simulink model "a2024_V2X_6V_Simulink_model"  (R2023b)
settings: Solver=VariableStepAuto  StartTime=0.0  StopTime=30  MaxStep=1e-2  RelTol=1e-3  AbsTol=1e-3
values from neighbouring files (symbols this model uses):
  b = 1.6    [a2024_v2x_matlab_6veh.m]
  mEgo = 1500    [a2024_v2x_matlab_6veh.m]
  Mode = 1    [a2024_v2x_matlab_6veh.m]    (also in v2x_matlab.m; v2x_matlabV2.m; v2x_matlab_6veh.m; v2x_matlab_R.m)
  pilot = (randi(s,[0 1],pilotsPerSym,1)-0.5)*2    [v2x_matlab.m]
  RxPowerV1 = zeros(sizeEgoWP+2, sizeV1WP+2)    [a2024_v2x_matlab_6veh.m]
  RxPowerV2 = zeros(sizeEgoWP+2, sizeV2WP+2)    [a2024_v2x_matlab_6veh.m]
  RxPowerV3 = zeros(sizeEgoWP+2, sizeV3WP+2)    [a2024_v2x_matlab_6veh.m]
  RxPowerV4 = zeros(sizeEgoWP+2, sizeV4WP+2)    [a2024_v2x_matlab_6veh.m]
  RxPowerV5 = zeros(sizeEgoWP+2, sizeV5WP+2)    [a2024_v2x_matlab_6veh.m]
  RxPowerV6 = zeros(sizeEgoWP+2, sizeV6WP+2)    [a2024_v2x_matlab_6veh.m]
  sampleTime = 0.1    [a2024_v2x_matlab_6veh.m]    (also in v2x_matlab.m; v2x_matlabV2.m; v2x_matlab_6veh.m; v2x_matlab_R.m)
  t_gap = 1.4    [a2024_v2x_matlab_6veh.m]
  waypoints = [egoWP(:,2) egoWP(:,1), zeroforwp]    [a2024_v2x_matlab_6veh.m]    (also in misc.m = data.data.ActorSpecifications(1,1).Waypoints(:,[1,2]); v2x_matlab.m = data.data.ActorSpecifications(1,1).Waypoints(:,[1,2]); v2x_matlabV2.m = [5 -1.6 0; v2x_matlab_R.m = [5 -1.6 0)
  ZeroActors = struct(     'ActorID',0,     'Position', [1000 1000 1000],      'Velocity', [0 0 0],      'Roll', 0,      'Pitch', 0,      'Yaw', 0,      'AngularVelocity', [0 0 0])    [v2x_matlabV2.m]    (also in v2x_matlab_R.m)
undefined symbols (not defined in the file or in its folder): driving, PredictionHorizon, Ts
libraries: commofdm x50, commcnvcod2 x39, simulink x34, commdigbbndam3 x31, commblkintrlv2 x26, commdigbbndpm3 x14, simulink_extras x12, drivingscenarioandsensors x3, mpcadaslib x2, commchan3 x1, vehdynlibdriver x1, commrandsrc3 x1
(part 1 of 6)
settings Model: DataDictionary=V2X.sldd  PacingRate=2  Creator=Fauszt Gábor  LastModifiedBy=Fauszt Gábor

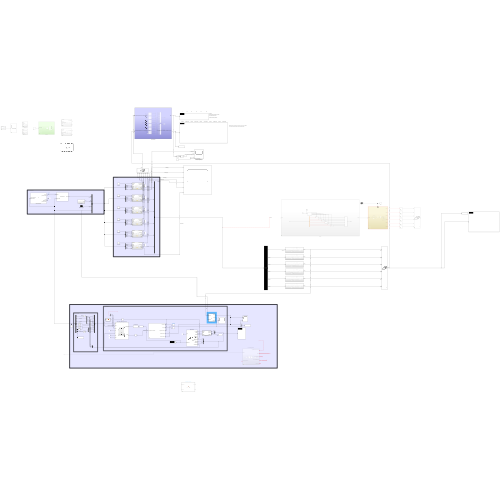
[thumbnail: Simulink's stored preview of the top-level diagram]
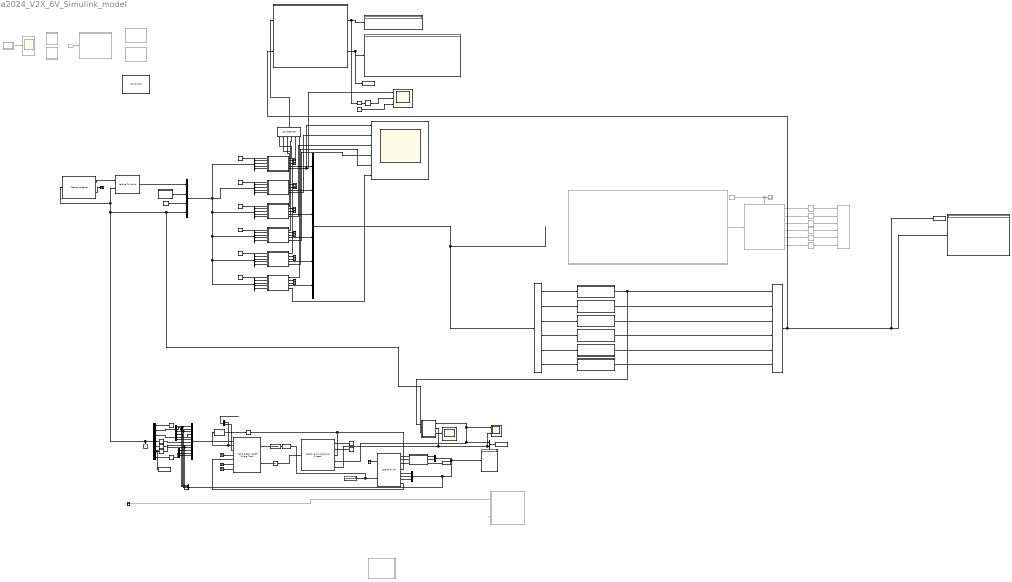
== system a2024_V2X_6V_Simulink_model ==
  note: ACC
  note: Display block can show only the first 10 columns of a matrix
      | thus, the columns of the 6th vehicle cannot be seen.
  note: V1 Received
  note: V1 Sent
  note: All packets sent' counter
  note: Received correct packets' counter
  note: PDR [%]
  note: V2
  note: V1
  note: Subsystem3
  note: Scenario Reader
  note: V3
  note: V4
  note: V5
  note: V6
  note: V2 Received
  note: V2 Sent
  note: V3 Received
  note: V3 Sent
  note: V4 Received
  note: V4 Sent
  note: V5 Received
  note: V5 Sent
  note: PDR of the last 20 packets
  note: Pack Ego Actor
  note: Ego Dynamics
  1/2 QPSK SNR és PDR a campus forgatókönyvre : Scope  NumInputPorts=3
  Adaptive Cruise Control System1 : mpcadaslib/Adaptive Cruise Control System  EgoModel=tf(1,[0.5,1,0])  InitialEgoVelocity=12  DefaultSpacing=0  MaxVelocity=20  MinAcceleration=-2  amin_ext=off  MaxAcceleration=4  amax_ext=off  Ts=0.01  PredictionHorizon=3  ControllerBehavior=0.950  suboptimal=off  maxiter=10  datatypeopt=double  optmode=off  trackmode=off
      settings: LibrarySourceBlock=mpclib/Automated Driving/Adaptive Cruise Control System
  Bus Creator : BusCreator  Inputs=6
  Bus Creator1 : BusCreator  Inputs=4
  Bus Creator2 : BusCreator  Inputs=4
  Bus Creator3 : BusCreator  Inputs=7  OutDataTypeStr=Bus: Actors
      settings: InheritFromInputs=off
  Bus Selector{,1..5} (6 alike) : BusSelector  OutputSignals=Trigger,Actors,Ego,Pilot
  Bus Selector6 : BusSelector  OutputSignals=Actor 1,Actor 2,Actor 3,Actor 4,Actor 5,Actor 6
  Bus Selector7 : BusSelector  OutputSignals=InertFrm.Cg.Disp.X,InertFrm.Cg.Disp.Y,InertFrm.Cg.Disp.Z,InertFrm.Cg.Vel.Xdot,InertFrm.Cg.Vel.Ydot,InertFrm.Cg.Vel.Zdot,InertFrm.Cg.Ang.phi,InertFrm.Cg.Ang.theta,InertFrm.Cg.Ang.psi,BdyFrm.Cg.AngVel.p,BdyFrm.Cg.AngVel.q,BdyFrm.Cg.AngVel.r
  Bus Selector8 : BusSelector  OutputSignals=X,Y,psi
  Bus Selector9 : BusSelector  OutputSignals=X,Y
  Calculate PDR : Subsystem
  Channel : Subsystem  Commented=on
  Clock : simulink_extras/Flip Flops/Clock  Commented=on  period=sampleTime/(6*6)
  Combo Box : ComboBox  LabelPosition=Hide
      settings: Values={{'64 QAM', '1/2 QPSK'}, [0 1]}
  Constant : Constant  Value=waypoints
  Constant1 : Constant  Value=13
  Constant2 : Constant  SampleTime=-1
  Constant3 : Constant  Value=12  VectorParams1D=off  SampleTime=sampleTime
  Constant4 : Constant  Value=t_gap  VectorParams1D=off  SampleTime=sampleTime
  Data Type Conversion : DataTypeConversion  SaturateOnIntegerOverflow=off  RndMeth=Floor
  Display{,1..4} (5 alike) : Display
  Ego trajectory : MATLAB Function  TreatAsAtomicUnit=on
  From1 : From  Commented=on
  Goto : Goto
  Integrator : Integrator
  Lane Keeping Assist : Subsystem  Commented=on
  Lateral Driver : vehdynlibdriver/Lateral Driver  extSteerOvr=off  extSteerHld=off  extSteerZero=off  steerOut=off  cntrlTypeLat=Stanley  coordMode=SAE J670 (Z-down)  angUnits=rad  tau=0.1  L=3  vecPose=off  dynamMode=on  PositionGainF=2.5  PositionGainR=2.5  YawRateGain=.2  DelayGain=.2  a=a  b=b  m=mEgo  Cy_f=Cy_f  Cy_r=70933  I=4013  Ksteer=18  theta=45*pi/180  aMode=2
  Low pass filter : TransferFcn  Denominator=[0.001 1]
  MATLAB Function : MATLAB Function  TreatAsAtomicUnit=on
  MATLAB Function1 : MATLAB Function  TreatAsAtomicUnit=on
  MATLAB Function2 : MATLAB Function  Commented=on  TreatAsAtomicUnit=on
  MATLAB Function3 : MATLAB Function  Commented=on  TreatAsAtomicUnit=on
  Matrix Concatenate : Concatenate  NumInputs=6  Mode=Multidimensional array  ConcatenateDimension=2
  Matrix Concatenate1 : Concatenate  Commented=on  NumInputs=6  Mode=Multidimensional array  ConcatenateDimension=2
  Matrix Concatenate2 : Concatenate  NumInputs=6  Mode=Multidimensional array  ConcatenateDimension=2
  Memory : Memory  InitialCondition=12
  MsgSendTrigger : simulink_extras/Flip Flops/Clock  period=0.1
  Mux : Mux  Inputs=3
  Mux1 : Mux  Inputs=3
  Mux2 : Mux  Inputs=3
  Pilot Port : Subsystem
  Queue : Subsystem  Commented=on
  Radians to Degrees{,1..3} (4 alike) : simulink_extras/Transformations/Radians to Degrees
  Rate Transition{1..6} (6 alike) : RateTransition  Commented=on  OutPortSampleTime=sampleTime/10
  Reshape : Reshape  OutputDimensionality=Customize  OutputDimensions=[24,1]
  Scenario Reader1 : drivingscenarioandsensors/Scenario Reader  ScenarioSource=From file  ScenarioFileName=C:\Users\Fauszt Gábor\Desktop\matlab\Fauszt_Gabor_matlab_v2x\v2.mat  ScenarioVariableName=scenario  OutputCoordinateSystem=Vehicle coordinates  EgoVehicleSource=Input port  EgoVehicleActorID=1  OrientVehiclesOnRoad=off  OutputEgoVehiclePose=on  OutputEgoVehicleState=off  SampleTime=sampleTime  LaneBoundaryOutput=All lane boundaries  LaneBoundaryDistance=0:0.5:9.5  LaneBoundaryLocation=Center of lane markings  BusNameSource=Auto  BusName=ActorsAll  BusNumActorsSource=Scenario  BusNumActors=100  BusName2Source=Auto  BusName2=BusLaneBoundaries  BusNumLaneBoundariesSource=Scenario  BusNumLaneBoundaries=10  BusName3Source=Auto  BusName3=BusEgoActor  BusName4Source=Auto  BusName4=BusEgoState  ShowCoordinateLabels=on  SimulateUsing=Interpreted execution
  Scope : Scope  NumInputPorts=6
  Scope1 : Scope
  Scope2 : Scope  NumInputPorts=2
  Scope3 : Scope  Commented=on
  Scope4 : Scope  Commented=on
  Selector : Selector  InputPortWidth=24  IndexOptions=Index vector (dialog)  Indices=4  OutputSizes=1
  Subsystem : Subsystem
  Subsystem1 : Subsystem  Commented=on
  Subsystem10 : Subsystem
  Subsystem11 : Subsystem
  Subsystem12 : Subsystem
  Subsystem13 : Subsystem
  Subsystem14 : Subsystem
  Subsystem2 : Subsystem  Commented=on
  Subsystem3 : Subsystem  Commented=on
  Subsystem4 : Subsystem
  Subsystem5 : Subsystem
  Subsystem6 : Subsystem
  Subsystem7 : Subsystem
  Subsystem8 : Subsystem
  Subsystem9 : Subsystem
  Terminator{,1..4,6..13,20..24} (18 alike) : Terminator
  To Workspace : ToWorkspace  VariableName=V6  SampleTime=-1
  To Workspace1 : ToWorkspace  VariableName=Compare_packets  SampleTime=-1
  To Workspace2 : ToWorkspace  VariableName=yaw  SampleTime=-1
  To Workspace3 : ToWorkspace  VariableName=RelVelPos  SampleTime=-1
  Vector Concatenate : Concatenate
  Vector Concatenate2 : Concatenate
  Vehicle 2 : Subsystem  Commented=on
  Vehicle 3 : Subsystem  Commented=on
  Vehicle Body 3DOF Single Track1 : autolibshared/Vehicle Body 3DOF Single Track  trackMode=Single (bicycle)  inputMode=External longitudinal velocity  frontSteerMode=on  rearSteerMode=off  windMode=off  muMode=off  extFMode=off  extMMode=off  htchFMode=off  htchMMode=off  extXo=off  extpsio=off  extxdoto=off  extro=off  extYo=off  extTamb=off  extydoto=off  aMode=2  NF=nrWheelsFr  NR=nrWheelsRe  m=mEgo  a=a  b=b  h=h  dh=1  hh=0.2  X_o=waypoints(1,1)  xdot_o=0  CalphaMode=off  sigmaMode=on  d=0  hl=0  w=[1.4,1.4]  Cy_f=Cy_f  Cy_r=Cy_r  sigma_f=sigma_f  sigma_r=sigma_r  alpha_f_brk=[-.1 .1]  Cy_f_data=[-9e3 9e3]  alpha_r_brk=[-.1 .1]  Cy_r_data=[-9e3 9e3]  Y_o=waypoints(1,2)  ydot_o=0  Izz=Izz  psi_o=3  r_o=0  Af=2  Cd=.3  Cl=.1  Cpm=.1  beta_w=[0 0.01:0.01:0.3]  Cs=[0 0.01:0.01:0.3]  Cym=[0 1e-6:0.01:0.3]  Pabs=101325  Tair=273  g=9.81  mu=1  xdot_tol=.01  Fznom=5000  Fxtire_sat=7e4  Fytire_sat=7e4  longOff=0  latOff=0  vertOff=0  wrapAng=off
  Vehicle To World : drivingscenarioandsensors/Vehicle To World  BusNameSource=Auto  BusName=ActorsaAll  SimulateUsing=Interpreted execution
  VehicleID : Constant
  VehicleID1 : Constant  Value=2
  VehicleID2 : Constant  Value=3
  VehicleID3 : Constant  Value=4
  VehicleID4 : Constant  Value=5
  VehicleID5 : Constant  Value=6
  wires:
  From1/1 -> Channel/1(EgoData)
  Scenario Reader1/2 -> Terminator/1
  VehicleID1/1 -> Subsystem4/1(VehicleID)
  VehicleID/1 -> Subsystem/1(VehicleID)
  VehicleID2/1 -> Subsystem5/1(VehicleID)
  Subsystem5/1(Sent packets) -> Matrix Concatenate/3
  MATLAB Function3/1(Dist) -> Scope4/1
  Subsystem3/3(Actor3) -> Rate Transition3/1
  Subsystem3/1(Actor1) -> Rate Transition1/1
  Subsystem3/4(Actor4) -> Rate Transition4/1
  VehicleID3/1 -> Subsystem6/1(VehicleID)
  VehicleID4/1 -> Subsystem7/1(VehicleID)
  Subsystem6/1(Sent packets) -> Matrix Concatenate/4
  Subsystem7/1(Sent packets) -> Matrix Concatenate/5
  Subsystem3/5(Actor5) -> Rate Transition5/1
  Lane Keeping Assist/1(Status) -> Terminator9/1
  Bus Creator3/1 -> Scenario Reader1/1, Vehicle To World/2, MATLAB Function/2(EgoActor), Bus Creator1/4, Goto/1  "Ego"
  VehicleID5/1 -> Subsystem8/1(VehicleID)
  Scenario Reader1/1 -> Vehicle To World/1
  Subsystem8/1(Sent packets) -> Matrix Concatenate/6
  Subsystem3/6(Actor6) -> Rate Transition6/1
  Clock/1 -> Scope3/1, Subsystem3/Enable
  Subsystem3/2(Actor2) -> Rate Transition2/1
  Subsystem/2(VehicleData) -> Terminator6/1
  Calculate PDR/1(PDR) -> Reshape/1, Display4/1
  Vehicle To World/1 -> Bus Creator1/1  "Actors"
  Subsystem/5(SNR) -> Scope/1, 1/2 QPSK SNR és PDR a campus forgatókönyvre/1  "V1 SNR [dB]"
  Subsystem/4(Actor1) -> Bus Creator/1  "Actor 1"
  Subsystem4/4(Actor2) -> Bus Creator/2  "Actor 2"
  Pilot Port/1(Pilot) -> Bus Creator1/2  "Pilot"
  MsgSendTrigger/1 -> Bus Creator1/3  "Trigger"
  Bus Selector/1 -> Subsystem/2(Trigger)  "<Trigger>"
  Bus Selector/2 -> Subsystem/3(Actors)  "<Actors>"
  Bus Selector/3 -> Subsystem/4(Ego)  "<Ego>"
  Bus Selector/4 -> Subsystem/5(Pilot)  "<Pilot>"
  Subsystem/3(V1) -> Terminator7/1  "V1"
  Subsystem4/2(VehicleData) -> Terminator8/1  "V2"
  Subsystem5/2(VehicleData) -> Terminator10/1  "V3"
  Subsystem6/2(VehicleData) -> Terminator11/1  "V4"
  Subsystem7/2(VehicleData) -> Terminator12/1  "V5"
  Subsystem8/2(VehicleData) -> Terminator13/1  "V6"
  Bus Selector1/2 -> Subsystem4/3(Actors)  "<Actors>"
  Bus Selector1/4 -> Subsystem4/5(Pilot)  "<Pilot>"
  Bus Selector1/3 -> Subsystem4/4(Ego)  "<Ego>"
  Bus Selector1/1 -> Subsystem4/2(Trigger)  "<Trigger>"
  Bus Selector2/4 -> Subsystem5/5(Pilot)  "<Pilot>"
  Bus Selector2/1 -> Subsystem5/2(Trigger)  "<Trigger>"
  Bus Selector2/3 -> Subsystem5/4(Ego)  "<Ego>"
  Bus Selector2/2 -> Subsystem5/3(Actors)  "<Actors>"
  Bus Selector3/3 -> Subsystem6/4(Ego)  "<Ego>"
  Bus Selector3/2 -> Subsystem6/3(Actors)  "<Actors>"
  Bus Selector3/4 -> Subsystem6/5(Pilot)  "<Pilot>"
  Bus Selector3/1 -> Subsystem6/2(Trigger)  "<Trigger>"
  Bus Selector4/3 -> Subsystem7/4(Ego)  "<Ego>"
  Bus Selector4/2 -> Subsystem7/3(Actors)  "<Actors>"
  Bus Selector4/4 -> Subsystem7/5(Pilot)  "<Pilot>"
  Bus Selector4/1 -> Subsystem7/2(Trigger)  "<Trigger>"
  Bus Selector5/1 -> Subsystem8/2(Trigger)  "<Trigger>"
  Bus Selector5/2 -> Subsystem8/3(Actors)  "<Actors>"
  Bus Selector5/3 -> Subsystem8/4(Ego)  "<Ego>"
  Bus Selector5/4 -> Subsystem8/5(Pilot)  "<Pilot>"
  Bus Creator1/1 -> Bus Selector5/1, Bus Selector4/1, Bus Selector3/1, Bus Selector2/1, Bus Selector/1, Bus Selector1/1
  Subsystem5/4(Actor3) -> Bus Creator/3  "Actor 3"
  Subsystem6/4(Actor4) -> Bus Creator/4  "Actor 4"
  Subsystem7/4(Actor5) -> Bus Creator/5  "Actor 5"
  Subsystem8/4(Actor6) -> Bus Creator/6  "Actor 6"
  Subsystem8/5(SNR) -> Scope/6  "V6 SNR [dB]"
  Subsystem7/5(SNR) -> Scope/5  "V5 SNR [dB]"
  Subsystem6/5(SNR) -> Scope/4  "V4 SNR [dB]"
  Subsystem5/5(SNR) -> Scope/3  "V3 SNR [dB]"
  Subsystem4/5(SNR) -> Scope/2  "V2 SNR [dB]"
  Subsystem/1(Sent packets) -> Matrix Concatenate/1
  Matrix Concatenate/1 -> Calculate PDR/1(Sent packets (Actors bus from Scenario Reader))
  Subsystem4/3(V2) -> Terminator20/1  "V1"
  Subsystem5/3(V3) -> Terminator21/1  "V1"
  Subsystem6/3(V4) -> Terminator22/1  "V1"
  Subsystem7/3(V5) -> Terminator23/1  "V1"
  Subsystem8/3(V6) -> Terminator24/1  "V1"
  Queue/1(Signal) -> Subsystem3/1(Signal)
  Bus Creator/1 -> Bus Selector6/1  "Actors"
  Calculate PDR/2(Sent and Received vectors side by side for comparison) -> Display3/1, To Workspace1/1
  Selector/1 -> 1/2 QPSK SNR és PDR a campus forgatókönyvre/2  "PDR az utolsó 10 csomagra [%]"
  Reshape/1 -> Selector/1
  Constant1/1 -> 1/2 QPSK SNR és PDR a campus forgatókönyvre/3  "Szabvány szerinti SNR határérték [dB]"
  Subsystem4/1(Sent packets) -> Matrix Concatenate/2
  Bus Selector6/1 -> Subsystem9/1(Inport)  "<Actor 1>"
  Subsystem9/1(Outport) -> MATLAB Function/1(V1Actor), Matrix Concatenate2/1
  Bus Selector6/3 -> Subsystem11/1(Inport)  "<Actor 3>"
  Bus Selector6/2 -> Subsystem10/1(Inport)  "<Actor 2>"
  Bus Selector6/4 -> Subsystem12/1(Inport)  "<Actor 4>"
  Bus Selector6/6 -> Subsystem14/1(Inport)  "<Actor 6>"
  Bus Selector6/5 -> Subsystem13/1(Inport)  "<Actor 5>"
  Subsystem10/1(Outport) -> Matrix Concatenate2/2
  Subsystem11/1(Outport) -> Matrix Concatenate2/3
  Subsystem12/1(Outport) -> Matrix Concatenate2/4
  Subsystem13/1(Outport) -> Matrix Concatenate2/5
  Subsystem14/1(Outport) -> Matrix Concatenate2/6
  Rate Transition4/1 -> Matrix Concatenate1/4
  Rate Transition2/1 -> Matrix Concatenate1/2
  Rate Transition6/1 -> Matrix Concatenate1/6
  Rate Transition1/1 -> Matrix Concatenate1/1
  Rate Transition3/1 -> Matrix Concatenate1/3
  Rate Transition5/1 -> Matrix Concatenate1/5
  ? -> Lane Keeping Assist/3(Lane Assist Offset)
  Constant4/1 -> Adaptive Cruise Control System1/2
  Ego trajectory/3(YawRef) -> Lateral Driver/3
  Constant3/1 -> Adaptive Cruise Control System1/1
  Vehicle Body 3DOF Single Track1/3 -> Vector Concatenate/2
  Bus Selector7/9 -> Radians to Degrees3/1, Bus Creator2/4  "<psi>"
  MATLAB Function1/1(y) -> Memory/1
  Mux/1 -> Radians to Degrees/1
  Bus Selector8/1 -> Lateral Driver/6  "<X>"
  Integrator/1 -> Vehicle Body 3DOF Single Track1/2
  Ego trajectory/1(LongRef) -> Lateral Driver/1
  Radians to Degrees3/1 -> To Workspace2/1, Bus Creator3/6
  Constant2/1 -> Bus Creator3/1  "ActorID"
  Ego trajectory/2(LatRef) -> Lateral Driver/2
  Vehicle Body 3DOF Single Track1/2 -> Vector Concatenate/1, MATLAB Function1/1(xdotin)  "Longitudinal velocity of ego"
  ? -> Lane Keeping Assist/1(Longitudinal velocity of ego)
  Bus Selector7/12 -> Mux/3  "<r>"
  Matrix Concatenate2/1 -> Display2/1, To Workspace/1, Calculate PDR/2(Received packets (Matrix from the processed data by ego))
  Lane Keeping Assist/2(SteeringAngle in rad) -> ?
  Mux1/1 -> Bus Creator3/2  "Position"
  Bus Selector7/6 -> Mux2/3  "<Zdot>"
  ? -> Lane Keeping Assist/2(Enable)
  Vehicle Body 3DOF Single Track1/4 -> Terminator2/1
  Bus Selector7/5 -> Mux2/1  "<Ydot>"
  Bus Selector7/10 -> Mux/1  "<p>"
  Bus Selector7/4 -> Mux2/2  "<Xdot>"
  Lateral Driver/2 -> Data Type Conversion/1, Display/1
  Vehicle Body 3DOF Single Track1/6 -> Terminator3/1
  Data Type Conversion/1 -> Low pass filter/1
  ? -> Lane Keeping Assist/4(lane boundaries Bus)
  Adaptive Cruise Control System1/1 -> Integrator/1  "Acceleration of ego"
  Radians to Degrees2/1 -> Bus Creator3/5
  Bus Selector7/3 -> Mux1/3, Bus Creator2/3  "<Z>"
  Vector Concatenate/1 -> ?
  Bus Selector9/1 -> Ego trajectory/1(EgoFdbX)  "<X>"
  ? -> Lane Keeping Assist/5(Driver Steer)
  Vector Concatenate2/1 -> To Workspace3/1
  Radians to Degrees1/1 -> Bus Creator3/4
  Memory/1 -> Lateral Driver/5, Adaptive Cruise Control System1/3
  Vehicle Body 3DOF Single Track1/5 -> Lateral Driver/9  "r"
  Vehicle Body 3DOF Single Track1/7 -> Terminator4/1
  Radians to Degrees/1 -> Bus Creator3/7  "AngularVelocity"
  Bus Selector7/8 -> Radians to Degrees2/1  "<theta>"
  Constant/1 -> Ego trajectory/3(waypoints)
  Low pass filter/1 -> Vehicle Body 3DOF Single Track1/1
  Bus Selector7/1 -> Mux1/2, Bus Creator2/1  "<X>"
  Bus Selector7/7 -> Radians to Degrees1/1  "<phi>"
  Vehicle Body 3DOF Single Track1/1 -> Bus Selector7/1
  Mux2/1 -> Bus Creator3/3  "Velocity"
  Bus Selector8/3 -> Lateral Driver/8  "<psi>"
  Bus Creator2/1 -> Bus Selector9/1, Display1/1, Bus Selector8/1
  Bus Selector7/11 -> Mux/2  "<q>"
  Bus Selector7/2 -> Mux1/1, Bus Creator2/2  "<Y>"
  Bus Selector8/2 -> Lateral Driver/7  "<Y>"
  Lateral Driver/1 -> Terminator1/1
  MATLAB Function/2(relVel) -> Scope2/2, Vector Concatenate2/2, Adaptive Cruise Control System1/5
  MATLAB Function/1(relDist) -> Adaptive Cruise Control System1/4, Vector Concatenate2/1, Scope2/1
  Bus Selector9/2 -> Ego trajectory/2(EgoFdbY)  "<Y>"
  MATLAB Function/3(EgoPos) -> Scope1/1

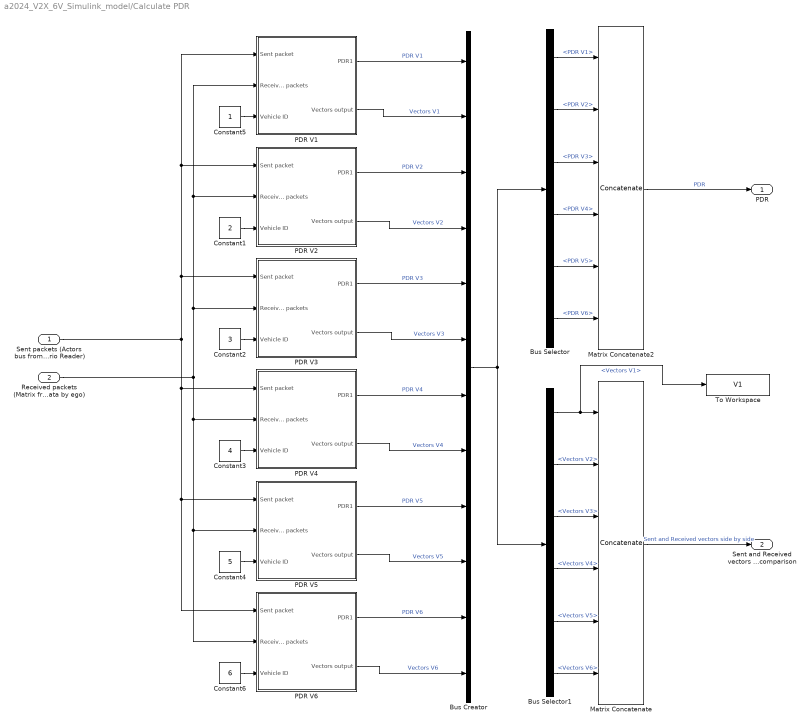
== system a2024_V2X_6V_Simulink_model/Calculate PDR ==
  Sent packets (Actors bus from Scenario Reader) : Inport
  Received packets (Matrix from the processed data by ego) : Inport  Port=2
  Bus Creator : BusCreator  Inputs=12
  Bus Selector : BusSelector  OutputSignals=PDR V1,PDR V2,PDR V3,PDR V4,PDR V5,PDR V6
  Bus Selector1 : BusSelector  OutputSignals=Vectors V1,Vectors V2,Vectors V3,Vectors V4,Vectors V5,Vectors V6
  Constant1 : Constant  Value=2  OutDataTypeStr=int16
  Constant2 : Constant  Value=3  OutDataTypeStr=int16
  Constant3 : Constant  Value=4  OutDataTypeStr=int16
  Constant4 : Constant  Value=5  OutDataTypeStr=int16
  Constant5 : Constant  OutDataTypeStr=int16
  Constant6 : Constant  Value=6  OutDataTypeStr=int16
  Matrix Concatenate : Concatenate  NumInputs=6  Mode=Multidimensional array  ConcatenateDimension=2
  Matrix Concatenate2 : Concatenate  NumInputs=6  Mode=Multidimensional array  ConcatenateDimension=2
  PDR V1 : Subsystem
  PDR V2 : Subsystem
  PDR V3 : Subsystem
  PDR V4 : Subsystem
  PDR V5 : Subsystem
  PDR V6 : Subsystem
  To Workspace : ToWorkspace  VariableName=V1  SampleTime=-1
  PDR : Outport
  Sent and Received vectors side by side for comparison : Outport  Port=2
  wires:
  Bus Selector1/6 -> Matrix Concatenate/6  "<Vectors V6>"
  Bus Creator/1 -> Bus Selector/1, Bus Selector1/1
  Bus Selector1/3 -> Matrix Concatenate/3  "<Vectors V3>"
  PDR V1/2(Vectors output) -> Bus Creator/2  "Vectors V1"
  Sent packets (Actors bus from Scenario Reader)/1 -> PDR V4/1(Sent packet), PDR V6/1(Sent packet), PDR V5/1(Sent packet), PDR V3/1(Sent packet), PDR V2/1(Sent packet), PDR V1/1(Sent packet)
  Received packets (Matrix from the processed data by ego)/1 -> PDR V4/2(Received packets), PDR V6/2(Received packets), PDR V5/2(Received packets), PDR V3/2(Received packets), PDR V2/2(Received packets), PDR V1/2(Received packets)
  PDR V5/1(PDR1) -> Bus Creator/9  "PDR V5"
  Matrix Concatenate/1 -> Sent and Received vectors side by side for comparison/1  "Sent and Received vectors side by side"
  Constant1/1 -> PDR V2/3(Vehicle ID)
  PDR V3/2(Vectors output) -> Bus Creator/6  "Vectors V3"
  Bus Selector/1 -> Matrix Concatenate2/1  "<PDR V1>"
  Bus Selector1/4 -> Matrix Concatenate/4  "<Vectors V4>"
  Constant4/1 -> PDR V5/3(Vehicle ID)
  Bus Selector/4 -> Matrix Concatenate2/4  "<PDR V4>"
  Bus Selector1/5 -> Matrix Concatenate/5  "<Vectors V5>"
  Bus Selector1/1 -> To Workspace/1, Matrix Concatenate/1  "<Vectors V1>"
  Bus Selector1/2 -> Matrix Concatenate/2  "<Vectors V2>"
  PDR V6/2(Vectors output) -> Bus Creator/12  "Vectors V6"
  Bus Selector/5 -> Matrix Concatenate2/5  "<PDR V5>"
  Constant3/1 -> PDR V4/3(Vehicle ID)
  PDR V2/2(Vectors output) -> Bus Creator/4  "Vectors V2"
  Constant6/1 -> PDR V6/3(Vehicle ID)
  Bus Selector/3 -> Matrix Concatenate2/3  "<PDR V3>"
  Bus Selector/6 -> Matrix Concatenate2/6  "<PDR V6>"
  Bus Selector/2 -> Matrix Concatenate2/2  "<PDR V2>"
  PDR V1/1(PDR1) -> Bus Creator/1  "PDR V1"
  Constant5/1 -> PDR V1/3(Vehicle ID)
  Constant2/1 -> PDR V3/3(Vehicle ID)
  PDR V5/2(Vectors output) -> Bus Creator/10  "Vectors V5"
  PDR V2/1(PDR1) -> Bus Creator/3  "PDR V2"
  PDR V3/1(PDR1) -> Bus Creator/5  "PDR V3"
  PDR V4/2(Vectors output) -> Bus Creator/8  "Vectors V4"
  PDR V4/1(PDR1) -> Bus Creator/7  "PDR V4"
  PDR V6/1(PDR1) -> Bus Creator/11  "PDR V6"
  Matrix Concatenate2/1 -> PDR/1  "PDR"

== system a2024_V2X_6V_Simulink_model/Channel ==
  EgoData : Inport
  AWGN Channel : commchan3/AWGN Channel  LegacyMode=off  NoiseMethod="Signal to noise ratio  (SNR)"  noiseMode="Signal to noise ratio  (SNR)"  EbNo=10  EsNo=10  SNR=60  BitsPerSymbol=1  SignalPower=1  SamplesPerSymbol=1  SymbolPeriod=1  VarianceSource=Parameter  Variance=1  RandomStream=Global stream  Seed=67  SimulateUsing=Interpreted execution
  Constant : Constant  Value=ZeroActors  OutDataTypeStr=Bus: Actors  SampleTime=sampleTime
  Constant1 : Constant  Commented=on  Value=randn(10)+55  SampleTime=sampleTime
  Entity Multicast : EntityMulticast  InputPortMessageModes=m  MulticastTag=B
  Entity Multicast1 : EntityMulticast  InputPortMessageModes=m  MulticastTag=B
  Entity Multicast2 : EntityMulticast  InputPortMessageModes=m  MulticastTag=B
  MATLAB Function1 : MATLAB Function  TreatAsAtomicUnit=on
  MATLAB Function4 : MATLAB Function  TreatAsAtomicUnit=on
  MATLAB Function9 : MATLAB Function  TreatAsAtomicUnit=on
  Multicast Receive Queue : Queue  OutputPortMessageModes=m  EntityArrivalSource=Multicast
  Receive : Receive  InputPortMessageModes=m  UseInternalQueue=off  QueueOverwriting=on  QueueLength=1  QueueType=LIFO
  Scope : Scope
  Send : Send  OutputPortMessageModes=m
  Send1 : Send  OutputPortMessageModes=m
  Send2 : Send  OutputPortMessageModes=m
  Terminator : Terminator
  wires:
  Multicast Receive Queue/1 -> Receive/1
  AWGN Channel/1 -> MATLAB Function1/1(ActorsIn)
  Receive/1 -> AWGN Channel/1
  MATLAB Function1/1(Actors) -> MATLAB Function9/2(Actors)
  MATLAB Function1/2(Positions) -> MATLAB Function9/3(Positions)  "Positions"
  Constant/1 -> MATLAB Function9/4(ZeroActors)
  MATLAB Function9/4(PSR) -> MATLAB Function4/1(PSR)
  MATLAB Function9/3(ThresholdActor) -> Send/1
  MATLAB Function9/2(InterferingActor) -> Send2/1
  MATLAB Function9/1(LeadActor) -> Send1/1
  EgoData/1 -> MATLAB Function9/1(Ego), MATLAB Function1/2(Ego)
  Constant1/1 -> ?
  MATLAB Function1/3(Distances) -> Terminator/1  "Distances"
  MATLAB Function4/1(CBR) -> Scope/1
  Send1/1 -> Entity Multicast2/1
  Send2/1 -> Entity Multicast1/1
  Send/1 -> Entity Multicast/1

== system a2024_V2X_6V_Simulink_model/Lane Keeping Assist ==
  Longitudinal velocity of ego : Inport
  Enable : Inport  Port=2
  Lane Assist Offset : Inport  Port=3
  lane boundaries Bus : Inport  Port=4
  Driver Steer : Inport  Port=5
  Abs : Abs  SaturateOnIntegerOverflow=off
  Estimate lane center : Subsystem
  Lane Keeping Assist System : mpcadaslib/Lane Keeping Assist System  ModelType=Use vehicle parameters  VehicleMass=mEgo  VehicleYawInertia=2875  LengthToFront=a  LengthToRear=b  FrontTireStiffness=Cy_f  RearTireStiffness=Cy_r  EgoModelMatrixA=[-4.4021 ,-12.4603;1.3913,-5.1868]  EgoModelMatrixB=[24.1270;15.8609]  EgoModelMatrixC=[1,0;0,1]  InitialLongVel=16  TransportLag=0  MinSteering=-0.5  umin_ext=off  MaxSteering=0.5  umax_ext=off  Ts=0.1  PredictionHorizon=5  ControllerBehavior=0.100  suboptimal=off  maxiter=10  datatypeopt=double  optmode=off  trackmode=off
      link override Longitudinal velocity must be positive: stopWhenAssertionFail=on
      settings: LibrarySourceBlock=mpclib/Automated Driving/Lane Keeping Assist System
  Pack to Custom Sensor Data Format : Subsystem
  Subsystem : Subsystem
  Subsystem2 : Subsystem
  Vision Detection Generator : drivingscenarioandsensors/Vision Detection Generator  SensorIndex=1  DetectorOutput=Lanes only  UpdateInterval=0.1  LaneUpdateInterval=0.1  SensorLocation=[ 1.9, 0 ]  Height=1.1  Yaw=0  Pitch=1  Roll=0  BusNameSource=Auto  BusName=BusObjectDetections  BusName2Source=Auto  BusName2=BusLaneDetections  MaxNumDetectionsSource=Property  MaxNumDetections=50  MaxNumLanesSource=Property  MaxNumLanes=30  DetectionCoordinates=Ego Cartesian  SimulateUsing=Interpreted execution  MaxRange=10  BoundingBoxAccuracy=5  ProcessNoiseIntensity=5  MaxSpeed=100  MaxAllowedOcclusion=0.5  MinObjectImageSize=[ 15, 15 ]  DetectionProbability=0.9  FalsePositivesPerImage=0.1  MinLaneImageSize=[ 20, 3 ]  LaneBoundaryAccuracy=3  HasNoise=on  InitialSeedSource=Repeatable  InitialSeed=0  UsedSeed=driving.internal.SimulinkUtilities.seedManager(gcb)  ActorProfilesSource=From Scenario Reader block  ActorProfilesParameters=driving.internal.ActorProfilesParameters  ActorProfilesExpression=struct( 'ClassID', 0, 'Length', 4.7, 'Width', 1.8, 'Height', 1.4, 'OriginOffset', [ -1.35, 0, 0 ] )  Intrinsics=driving.internal.cameraIntrinsics('FocalLength',[1, 1 ])
  Status : Outport
  SteeringAngle in rad : Outport  Port=2
  wires:
  Subsystem/1(Departure Detected) -> Subsystem2/2(Set)
  Estimate lane center/2(Lateral Offset) -> Lane Keeping Assist System/3
  Enable/1 -> Subsystem2/1(Enable)
  Pack to Custom Sensor Data Format/1(lanes) -> Subsystem/2(Lane Sensor data), Estimate lane center/2(Lane Boundaries)
  Estimate lane center/1(Previewed Curvature) -> Lane Keeping Assist System/1
  Estimate lane center/3(Heading Angle) -> Lane Keeping Assist System/4
  lane boundaries Bus/1 -> Vision Detection Generator/1
  Vision Detection Generator/1 -> Pack to Custom Sensor Data Format/1(lane Detections)
  Lane Assist Offset/1 -> Subsystem/1(Lane Assist Offset)
  Driver Steer/1 -> Subsystem2/4(Driver Steer)
  Subsystem2/1(Status) -> Status/1
  Longitudinal velocity of ego/1 -> Abs/1, Estimate lane center/1(Longitudinal velocity of ego)
  Abs/1 -> Lane Keeping Assist System/2
  Subsystem2/2(SteeringAngle in rad) -> SteeringAngle in rad/1
  Lane Keeping Assist System/1 -> Subsystem2/3(Assisted Steer)  "Assisted Steer"

== system a2024_V2X_6V_Simulink_model/Pilot Port ==
  BPSK Modulator Baseband : commdigbbndpm3/BPSK Modulator Baseband  Ph=0  outDtype=double  outWordLen=16  outUDDataType=sfix(16)  outFracLenMode=Best precision  outFracLen=15  outDataTypeStr=double  outLastDataTypeStr=double
      settings: LibrarySourceBlock=|
      | commhdldigbbndpm/BPSK
      | Modulator
      | Baseband
  Bernoulli Binary Generator : commrandsrc3/Bernoulli Binary Generator  ProbabilityOfZero=0.5  SeedSource=Auto  Seed=0  SampleTime=0.01  SamplesPerFrame=4  OutputDataType=double  SimulateUsing=Interpreted execution
  Constant : Constant  Commented=on  Value=pilot
  Display : Display
  Rectangular QAM Modulator Baseband : commdigbbndam3/Rectangular QAM Modulator Baseband  Commented=on  M=2^6  InType=Integer  Enc=Gray  Mapping=[0:15]  PowType=Average Power  MinDist=2  AvgPow=1  PeakPow=1  Ph=0  outDtype=double  outWordLen=16  outUDDataType=sfix(16)  outFracLenMode=Best precision  outFracLen=15  outDataTypeStr=double  outLastDataTypeStr=double
      settings: LibrarySourceBlock=|
      | commhdldigbbndam/Rectangular QAM
      | Modulator
      | Baseband
  Reshape : Reshape  OutputDimensionality=Customize  OutputDimensions=[4,1]
  Pilot : Outport
  wires:
  Bernoulli Binary Generator/1 -> BPSK Modulator Baseband/1
  BPSK Modulator Baseband/1 -> Display/1, Reshape/1
  Reshape/1 -> Pilot/1

== system a2024_V2X_6V_Simulink_model/Queue ==
  Actors : Inport
  Bus Selector6 : BusSelector  OutputSignals=Actor 1,Actor 2,Actor 3,Actor 4,Actor 5,Actor 6
  Counter Limited : simulink/Sources/Counter Limited  uplimit=5  tsamp=sampleTime/(6*6)
  Merge : Merge  Inputs=6
  Scope1 : Scope
  Switch Case : SwitchCase  CaseConditions={0,1,2,3,4,5}  ShowDefaultCase=off
  Switch Case Action Subsystem : Subsystem  TreatAsAtomicUnit=on
  Switch Case Action Subsystem1 : Subsystem  TreatAsAtomicUnit=on
  Switch Case Action Subsystem2 : Subsystem  TreatAsAtomicUnit=on
  Switch Case Action Subsystem3 : Subsystem  TreatAsAtomicUnit=on
  Switch Case Action Subsystem4 : Subsystem  TreatAsAtomicUnit=on
  Switch Case Action Subsystem5 : Subsystem  TreatAsAtomicUnit=on
  Signal : Outport
  wires:
  Switch Case Action Subsystem2/1(Out1) -> Merge/3
  Counter Limited/1 -> Switch Case/1, Scope1/1  "Control"
  Switch Case Action Subsystem1/1(Out1) -> Merge/2
  Switch Case/2 -> Switch Case Action Subsystem1/Action
  Switch Case/1 -> Switch Case Action Subsystem/Action
  Switch Case Action Subsystem/1(Out1) -> Merge/1
  Bus Selector6/1 -> Switch Case Action Subsystem/1(Actor1)  "<Actor 1>"
  Bus Selector6/3 -> Switch Case Action Subsystem2/1(Actor1)  "<Actor 3>"
  Bus Selector6/2 -> Switch Case Action Subsystem1/1(Actor1)  "<Actor 2>"
  Switch Case Action Subsystem3/1(Out1) -> Merge/4
  Bus Selector6/6 -> Switch Case Action Subsystem5/1(Actor1)  "<Actor 6>"
  Switch Case/4 -> Switch Case Action Subsystem3/Action
  Bus Selector6/4 -> Switch Case Action Subsystem3/1(Actor1)  "<Actor 4>"
  Switch Case/5 -> Switch Case Action Subsystem4/Action
  Switch Case/6 -> Switch Case Action Subsystem5/Action
  Switch Case Action Subsystem5/1(Out1) -> Merge/6
  Switch Case Action Subsystem4/1(Out1) -> Merge/5
  Bus Selector6/5 -> Switch Case Action Subsystem4/1(Actor1)  "<Actor 5>"
  Switch Case/3 -> Switch Case Action Subsystem2/Action
  Actors/1 -> Bus Selector6/1
  Merge/1 -> Signal/1

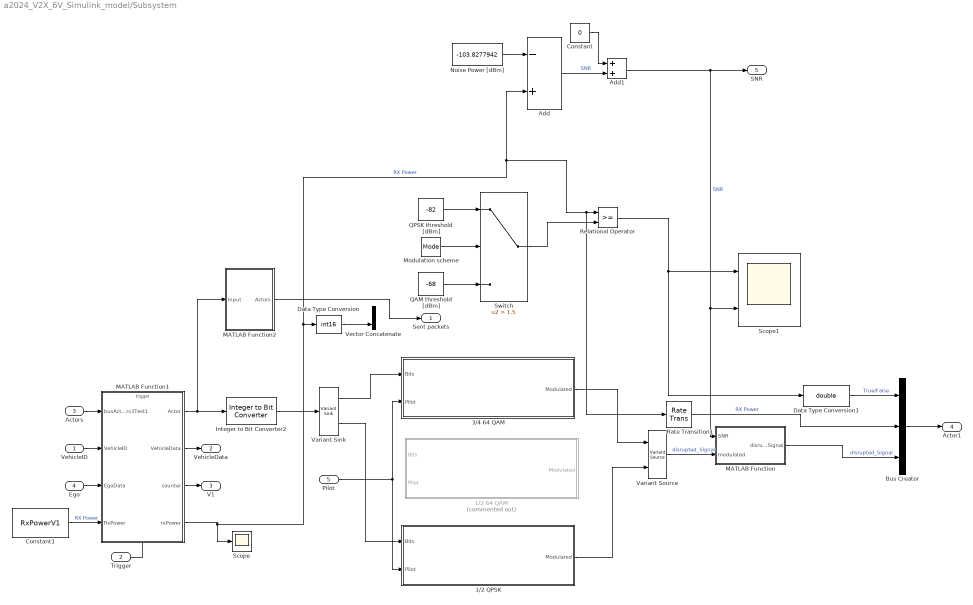
== system a2024_V2X_6V_Simulink_model/Subsystem ==
  VehicleID : Inport
  Trigger : Inport  Port=2
  Actors : Inport  Port=3
  Ego : Inport  Port=4
  Pilot : Inport  Port=5
  1/2 64 QAM : Subsystem  Commented=on  TreatAsAtomicUnit=on
  1/2 QPSK : Subsystem  TreatAsAtomicUnit=on
  3/4 64 QAM : Subsystem  TreatAsAtomicUnit=on
  Add : Sum  Inputs=-+
  Add1 : Sum
  Bus Creator : BusCreator  Inputs=3
  Constant : Constant  Value=0
  Constant1 : Constant  Value=RxPowerV1
  Data Type Conversion : DataTypeConversion  OutDataTypeStr=int16  SaturateOnIntegerOverflow=off  RndMeth=Floor
  Data Type Conversion1 : DataTypeConversion  OutDataTypeStr=double  SaturateOnIntegerOverflow=off  RndMeth=Floor
  Integer to Bit Converter2 : simulink/Logic and Bit Operations/Integer to Bit Converter  nbits=16  signedInputValues=Signed  bitOrder=MSB first  outDtype=boolean
  MATLAB Function : MATLAB Function  TreatAsAtomicUnit=on
  MATLAB Function1 : MATLAB Function  TreatAsAtomicUnit=on
  MATLAB Function2 : MATLAB Function  TreatAsAtomicUnit=on  SystemSampleTime=0.01
  Modulation scheme : Constant  Value=Mode
  Noise Power [dBm] : Constant  Value=-103.8277942
  QAM threshold [dBm] : Constant  Value=-68
  QPSK threshold [dBm] : Constant  Value=-82
  Rate Transition1 : RateTransition  OutPortSampleTime=sampleTime/10
  Relational Operator : RelationalOperator  OutDataTypeStr=boolean  RndMeth=Simplest  InputSameDT=off
  Scope : Scope
  Scope1 : Scope  NumInputPorts=2
  Switch : Switch  Criteria=u2 > Threshold  Threshold=1.5  SaturateOnIntegerOverflow=off  InputSameDT=off
  Variant Sink : VariantSink
  Variant Source : VariantSource
  Vector Concatenate : Concatenate
  Sent packets : Outport
  VehicleData : Outport  Port=2
  V1 : Outport  Port=3
  Actor1 : Outport  Port=4
  SNR : Outport  Port=5
  wires:
  MATLAB Function1/1(Actor) -> MATLAB Function2/1(input), Integer to Bit Converter2/1
  Ego/1 -> MATLAB Function1/3(EgoData)
  Actors/1 -> MATLAB Function1/1(busActors3Test1)
  VehicleID/1 -> MATLAB Function1/2(VehicleID)
  MATLAB Function1/2(VehicleData) -> VehicleData/1
  MATLAB Function1/3(counter) -> V1/1
  Trigger/1 -> MATLAB Function1/Trigger
  Integer to Bit Converter2/1 -> Variant Sink/1
  Pilot/1 -> 1/2 QPSK/2(Pilot), 3/4 64 QAM/2(Pilot)
  3/4 64 QAM/1(Modulated) -> Variant Source/1
  1/2 QPSK/1(Modulated) -> Variant Source/2
  Variant Sink/1 -> 3/4 64 QAM/1(Bits)
  Variant Sink/2 -> 1/2 QPSK/1(Bits)
  Noise Power [dBm]/1 -> Add/1
  QPSK threshold [dBm]/1 -> Switch/1
  QAM threshold [dBm]/1 -> Switch/3
  Modulation scheme/1 -> Switch/2
  Add1/1 -> MATLAB Function/1(SNR), Scope1/2, SNR/1  "SNR"
  Switch/1 -> Relational Operator/2
  Relational Operator/1 -> Data Type Conversion1/1, Scope1/1
  MATLAB Function1/4(rxPower) -> Scope/1, Data Type Conversion/1, Rate Transition1/1, Relational Operator/1, Add/2  "RX Power"
  Constant1/1 -> MATLAB Function1/4(RxPower)  "RX Power"
  Bus Creator/1 -> Actor1/1
  MATLAB Function2/1(Actors) -> Sent packets/1
  MATLAB Function/1(disrupted_Signal) -> Bus Creator/3  "disrupted_Signal"
  Data Type Conversion/1 -> Vector Concatenate/2
  Data Type Conversion1/1 -> Bus Creator/1  "True/False"
  Rate Transition1/1 -> Bus Creator/2  "RX Power"
  Variant Source/1 -> MATLAB Function/2(modulated)  "disrupted_Signal"
  Add/1 -> Add1/2  "SNR"
  Constant/1 -> Add1/1

== system a2024_V2X_6V_Simulink_model/Subsystem1 ==
  VehicleID : Inport
  Trigger : Inport  Port=2
  busActors3Test1 : Inport  Port=3
  Pilot : Inport  Port=4
  Actors : Inport  Port=5
  Constant2 : Constant  Value=[zeros(19,1)']  SampleTime=-1
  Entity Multicast1 : EntityMulticast  InputPortMessageModes=m
  Integer to Bit Converter2 : simulink/Logic and Bit Operations/Integer to Bit Converter  nbits=16  signedInputValues=Signed  bitOrder=MSB first  outDtype=boolean
  MATLAB Function1 : MATLAB Function  TreatAsAtomicUnit=on
  OFDM Modulator : commofdm/OFDM Modulator  StatePerturbationForJacobian=1.0e-05  FFTLength=64  NumGuardBandCarriers=[0;0]  InsertDCNull=on  PilotInputPort=on  PilotCarrierIndices=[12; 26; 40; 54]  CyclicPrefixLength=32  Windowing=off  WindowLength=16  OversamplingFactor=3  NumSymbols=1  NumTransmitAntennas=1  SimulateUsing=Interpreted execution
  Rectangular QAM Modulator Baseband2 : commdigbbndam3/Rectangular QAM Modulator Baseband  M=2^6  InType=Bit  Enc=Binary  Mapping=[0:15]  PowType=Average Power  MinDist=2  AvgPow=P_Signal  PeakPow=1  Ph=0  outDtype=double  outWordLen=16  outUDDataType=sfix(16)  outFracLenMode=Best precision  outFracLen=15  outDataTypeStr=double  outLastDataTypeStr=double
      settings: LibrarySourceBlock=|
      | commhdldigbbndam/Rectangular QAM
      | Modulator
      | Baseband
  Send1 : Send  OutputPortMessageModes=m
  Vector Concatenate : Concatenate
  VehicleData : Outport
  V2 : Outport  Port=2
  wires:
  MATLAB Function1/3(counter) -> V2/1
  MATLAB Function1/2(VehicleData) -> VehicleData/1
  Pilot/1 -> OFDM Modulator/2
  VehicleID/1 -> MATLAB Function1/2(VehicleID)
  busActors3Test1/1 -> MATLAB Function1/1(busActors3Test1)
  Trigger/1 -> MATLAB Function1/Trigger
  Integer to Bit Converter2/1 -> Rectangular QAM Modulator Baseband2/1
  OFDM Modulator/1 -> Send1/1  "OFDM modulated"
  Actors/1 -> MATLAB Function1/3(EgoData)
  Constant2/1 -> Vector Concatenate/2
  Rectangular QAM Modulator Baseband2/1 -> Vector Concatenate/1
  Send1/1 -> Entity Multicast1/1
  Vector Concatenate/1 -> OFDM Modulator/1  "After QAM Mod"
  MATLAB Function1/1(Actor) -> Integer to Bit Converter2/1

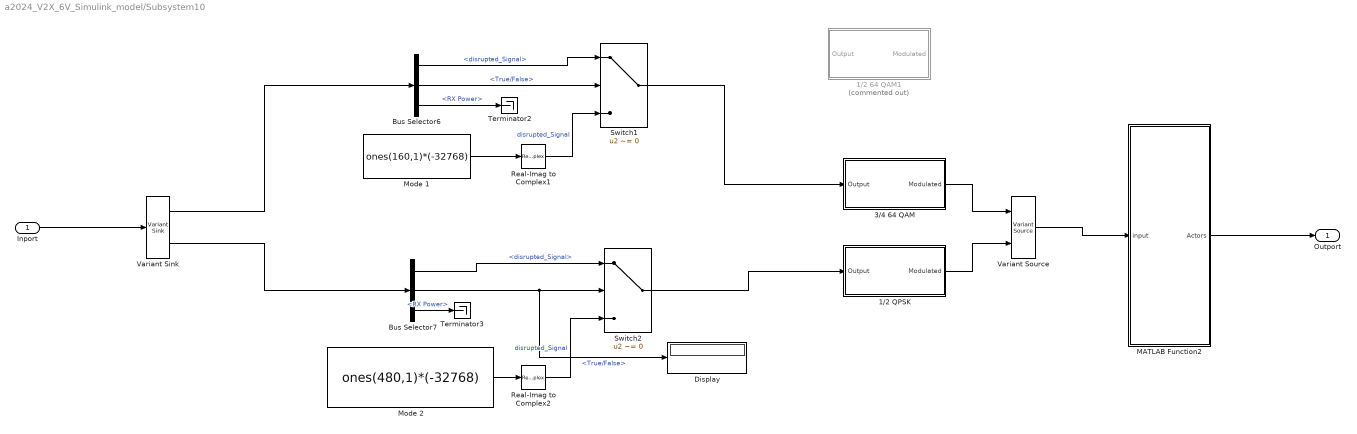
== system a2024_V2X_6V_Simulink_model/Subsystem10 ==
  Inport : Inport
  1/2 64 QAM1 : Subsystem  Commented=on  TreatAsAtomicUnit=on
  1/2 QPSK : Subsystem  TreatAsAtomicUnit=on
  3/4 64 QAM : Subsystem  TreatAsAtomicUnit=on
  Bus Selector6 : BusSelector  OutputSignals=disrupted_Signal,True/False,RX Power
  Bus Selector7 : BusSelector  OutputSignals=disrupted_Signal,True/False,RX Power
  Display : Display
  MATLAB Function2 : MATLAB Function  TreatAsAtomicUnit=on  SystemSampleTime=0.01
  Mode 1 : Constant  Value=ones(160,1)*(-32768)  OutDataTypeStr=Inherit: Inherit via back propagation
  Mode 2 : Constant  Value=ones(480,1)*(-32768)  OutDataTypeStr=Inherit: Inherit via back propagation
  Real-Imag to Complex1 : RealImagToComplex  Input=Real
  Real-Imag to Complex2 : RealImagToComplex  Input=Real
  Switch1 : Switch  Criteria=u2 ~= 0  OutDataTypeStr=double  SaturateOnIntegerOverflow=off  InputSameDT=off
  Switch2 : Switch  Criteria=u2 ~= 0  OutDataTypeStr=double  SaturateOnIntegerOverflow=off  InputSameDT=off
  Terminator2 : Terminator
  Terminator3 : Terminator
  Variant Sink : VariantSink
  Variant Source : VariantSource
  Outport : Outport
  wires:
  Mode 1/1 -> Real-Imag to Complex1/1
  Bus Selector7/1 -> Switch2/1  "<disrupted_Signal>"
  Switch2/1 -> 1/2 QPSK/1(Output)
  Bus Selector7/3 -> Terminator3/1  "<RX Power>"
  Switch1/1 -> 3/4 64 QAM/1(Output)
  Bus Selector7/2 -> Switch2/2, Display/1  "<True/False>"
  3/4 64 QAM/1(Modulated) -> Variant Source/1
  Bus Selector6/3 -> Terminator2/1  "<RX Power>"
  Bus Selector6/2 -> Switch1/2  "<True/False>"
  Mode 2/1 -> Real-Imag to Complex2/1
  Variant Sink/2 -> Bus Selector7/1
  Real-Imag to Complex2/1 -> Switch2/3  "disrupted_Signal"
  Variant Sink/1 -> Bus Selector6/1
  MATLAB Function2/1(Actors) -> Outport/1
  Inport/1 -> Variant Sink/1
  1/2 QPSK/1(Modulated) -> Variant Source/2
  Bus Selector6/1 -> Switch1/1  "<disrupted_Signal>"
  Variant Source/1 -> MATLAB Function2/1(input)
  Real-Imag to Complex1/1 -> Switch1/3  "disrupted_Signal"

== system a2024_V2X_6V_Simulink_model/Subsystem11 ==
  Inport : Inport
  1/2 64 QAM1 : Subsystem  Commented=on  TreatAsAtomicUnit=on
  1/2 QPSK : Subsystem  TreatAsAtomicUnit=on
  3/4 64 QAM : Subsystem  TreatAsAtomicUnit=on
  Bus Selector6 : BusSelector  OutputSignals=disrupted_Signal,True/False,RX Power
  Bus Selector7 : BusSelector  OutputSignals=disrupted_Signal,True/False,RX Power
  Display : Display
  MATLAB Function2 : MATLAB Function  TreatAsAtomicUnit=on  SystemSampleTime=0.01
  Mode 1 : Constant  Value=ones(160,1)*(-32768)  OutDataTypeStr=Inherit: Inherit via back propagation
  Mode 2 : Constant  Value=ones(480,1)*(-32768)  OutDataTypeStr=Inherit: Inherit via back propagation
  Real-Imag to Complex1 : RealImagToComplex  Input=Real
  Real-Imag to Complex2 : RealImagToComplex  Input=Real
  Switch1 : Switch  Criteria=u2 ~= 0  OutDataTypeStr=double  SaturateOnIntegerOverflow=off  InputSameDT=off
  Switch2 : Switch  Criteria=u2 ~= 0  OutDataTypeStr=double  SaturateOnIntegerOverflow=off  InputSameDT=off
  Terminator2 : Terminator
  Terminator3 : Terminator
  Variant Sink : VariantSink
  Variant Source : VariantSource
  Outport : Outport
  wires:
  Real-Imag to Complex1/1 -> Switch1/3  "disrupted_Signal"
  Variant Source/1 -> MATLAB Function2/1(input)
  Bus Selector6/1 -> Switch1/1  "<disrupted_Signal>"
  1/2 QPSK/1(Modulated) -> Variant Source/2
  Inport/1 -> Variant Sink/1
  MATLAB Function2/1(Actors) -> Outport/1
  Variant Sink/1 -> Bus Selector6/1
  Real-Imag to Complex2/1 -> Switch2/3  "disrupted_Signal"
  Variant Sink/2 -> Bus Selector7/1
  Mode 2/1 -> Real-Imag to Complex2/1
  Bus Selector6/2 -> Switch1/2  "<True/False>"
  Bus Selector6/3 -> Terminator2/1  "<RX Power>"
  3/4 64 QAM/1(Modulated) -> Variant Source/1
  Bus Selector7/2 -> Display/1, Switch2/2  "<True/False>"
  Switch1/1 -> 3/4 64 QAM/1(Output)
  Bus Selector7/3 -> Terminator3/1  "<RX Power>"
  Switch2/1 -> 1/2 QPSK/1(Output)
  Bus Selector7/1 -> Switch2/1  "<disrupted_Signal>"
  Mode 1/1 -> Real-Imag to Complex1/1

== system a2024_V2X_6V_Simulink_model/Subsystem12 ==
  Inport : Inport
  1/2 64 QAM1 : Subsystem  Commented=on  TreatAsAtomicUnit=on
  1/2 QPSK : Subsystem  TreatAsAtomicUnit=on
  3/4 64 QAM : Subsystem  TreatAsAtomicUnit=on
  Bus Selector6 : BusSelector  OutputSignals=disrupted_Signal,True/False,RX Power
  Bus Selector7 : BusSelector  OutputSignals=disrupted_Signal,True/False,RX Power
  Display : Display
  MATLAB Function2 : MATLAB Function  TreatAsAtomicUnit=on  SystemSampleTime=0.01
  Mode 1 : Constant  Value=ones(160,1)*(-32768)  OutDataTypeStr=Inherit: Inherit via back propagation
  Mode 2 : Constant  Value=ones(480,1)*(-32768)  OutDataTypeStr=Inherit: Inherit via back propagation
  Real-Imag to Complex1 : RealImagToComplex  Input=Real
  Real-Imag to Complex2 : RealImagToComplex  Input=Real
  Switch1 : Switch  Criteria=u2 ~= 0  OutDataTypeStr=double  SaturateOnIntegerOverflow=off  InputSameDT=off
  Switch2 : Switch  Criteria=u2 ~= 0  OutDataTypeStr=double  SaturateOnIntegerOverflow=off  InputSameDT=off
  Terminator2 : Terminator
  Terminator3 : Terminator
  Variant Sink : VariantSink
  Variant Source : VariantSource
  Outport : Outport
  wires:
  Mode 1/1 -> Real-Imag to Complex1/1
  Bus Selector7/1 -> Switch2/1  "<disrupted_Signal>"
  Switch2/1 -> 1/2 QPSK/1(Output)
  Bus Selector7/3 -> Terminator3/1  "<RX Power>"
  Switch1/1 -> 3/4 64 QAM/1(Output)
  Bus Selector7/2 -> Switch2/2, Display/1  "<True/False>"
  3/4 64 QAM/1(Modulated) -> Variant Source/1
  Bus Selector6/3 -> Terminator2/1  "<RX Power>"
  Bus Selector6/2 -> Switch1/2  "<True/False>"
  Mode 2/1 -> Real-Imag to Complex2/1
  Variant Sink/2 -> Bus Selector7/1
  Real-Imag to Complex2/1 -> Switch2/3  "disrupted_Signal"
  Variant Sink/1 -> Bus Selector6/1
  MATLAB Function2/1(Actors) -> Outport/1
  Inport/1 -> Variant Sink/1
  1/2 QPSK/1(Modulated) -> Variant Source/2
  Bus Selector6/1 -> Switch1/1  "<disrupted_Signal>"
  Variant Source/1 -> MATLAB Function2/1(input)
  Real-Imag to Complex1/1 -> Switch1/3  "disrupted_Signal"

== system a2024_V2X_6V_Simulink_model/Subsystem13 ==
  Inport : Inport
  1/2 64 QAM1 : Subsystem  Commented=on  TreatAsAtomicUnit=on
  1/2 QPSK : Subsystem  TreatAsAtomicUnit=on
  3/4 64 QAM : Subsystem  TreatAsAtomicUnit=on
  Bus Selector6 : BusSelector  OutputSignals=disrupted_Signal,True/False,RX Power
  Bus Selector7 : BusSelector  OutputSignals=disrupted_Signal,True/False,RX Power
  Display : Display
  MATLAB Function2 : MATLAB Function  TreatAsAtomicUnit=on  SystemSampleTime=0.01
  Mode 1 : Constant  Value=ones(160,1)*(-32768)  OutDataTypeStr=Inherit: Inherit via back propagation
  Mode 2 : Constant  Value=ones(480,1)*(-32768)  OutDataTypeStr=Inherit: Inherit via back propagation
  Real-Imag to Complex1 : RealImagToComplex  Input=Real
  Real-Imag to Complex2 : RealImagToComplex  Input=Real
  Switch1 : Switch  Criteria=u2 ~= 0  OutDataTypeStr=double  SaturateOnIntegerOverflow=off  InputSameDT=off
  Switch2 : Switch  Criteria=u2 ~= 0  OutDataTypeStr=double  SaturateOnIntegerOverflow=off  InputSameDT=off
  Terminator2 : Terminator
  Terminator3 : Terminator
  Variant Sink : VariantSink
  Variant Source : VariantSource
  Outport : Outport
  wires:
  Real-Imag to Complex1/1 -> Switch1/3  "disrupted_Signal"
  Variant Source/1 -> MATLAB Function2/1(input)
  Bus Selector6/1 -> Switch1/1  "<disrupted_Signal>"
  1/2 QPSK/1(Modulated) -> Variant Source/2
  Inport/1 -> Variant Sink/1
  MATLAB Function2/1(Actors) -> Outport/1
  Variant Sink/1 -> Bus Selector6/1
  Real-Imag to Complex2/1 -> Switch2/3  "disrupted_Signal"
  Variant Sink/2 -> Bus Selector7/1
  Mode 2/1 -> Real-Imag to Complex2/1
  Bus Selector6/2 -> Switch1/2  "<True/False>"
  Bus Selector6/3 -> Terminator2/1  "<RX Power>"
  3/4 64 QAM/1(Modulated) -> Variant Source/1
  Bus Selector7/2 -> Display/1, Switch2/2  "<True/False>"
  Switch1/1 -> 3/4 64 QAM/1(Output)
  Bus Selector7/3 -> Terminator3/1  "<RX Power>"
  Switch2/1 -> 1/2 QPSK/1(Output)
  Bus Selector7/1 -> Switch2/1  "<disrupted_Signal>"
  Mode 1/1 -> Real-Imag to Complex1/1

== system a2024_V2X_6V_Simulink_model/Subsystem14 ==
  Inport : Inport
  1/2 64 QAM1 : Subsystem  Commented=on  TreatAsAtomicUnit=on
  1/2 QPSK : Subsystem  TreatAsAtomicUnit=on
  3/4 64 QAM : Subsystem  TreatAsAtomicUnit=on
  Bus Selector6 : BusSelector  OutputSignals=disrupted_Signal,True/False,RX Power
  Bus Selector7 : BusSelector  OutputSignals=disrupted_Signal,True/False,RX Power
  Display : Display
  MATLAB Function2 : MATLAB Function  TreatAsAtomicUnit=on  SystemSampleTime=0.01
  Mode 1 : Constant  Value=ones(160,1)*(-32768)  OutDataTypeStr=Inherit: Inherit via back propagation
  Mode 2 : Constant  Value=ones(480,1)*(-32768)  OutDataTypeStr=Inherit: Inherit via back propagation
  Real-Imag to Complex1 : RealImagToComplex  Input=Real
  Real-Imag to Complex2 : RealImagToComplex  Input=Real
  Switch1 : Switch  Criteria=u2 ~= 0  OutDataTypeStr=double  SaturateOnIntegerOverflow=off  InputSameDT=off
  Switch2 : Switch  Criteria=u2 ~= 0  OutDataTypeStr=double  SaturateOnIntegerOverflow=off  InputSameDT=off
  Terminator2 : Terminator
  Terminator3 : Terminator
  Variant Sink : VariantSink
  Variant Source : VariantSource
  Outport : Outport
  wires:
  Mode 1/1 -> Real-Imag to Complex1/1
  Bus Selector7/1 -> Switch2/1  "<disrupted_Signal>"
  Switch2/1 -> 1/2 QPSK/1(Output)
  Bus Selector7/3 -> Terminator3/1  "<RX Power>"
  Switch1/1 -> 3/4 64 QAM/1(Output)
  Bus Selector7/2 -> Switch2/2, Display/1  "<True/False>"
  3/4 64 QAM/1(Modulated) -> Variant Source/1
  Bus Selector6/3 -> Terminator2/1  "<RX Power>"
  Bus Selector6/2 -> Switch1/2  "<True/False>"
  Mode 2/1 -> Real-Imag to Complex2/1
  Variant Sink/2 -> Bus Selector7/1
  Real-Imag to Complex2/1 -> Switch2/3  "disrupted_Signal"
  Variant Sink/1 -> Bus Selector6/1
  MATLAB Function2/1(Actors) -> Outport/1
  Inport/1 -> Variant Sink/1
  1/2 QPSK/1(Modulated) -> Variant Source/2
  Bus Selector6/1 -> Switch1/1  "<disrupted_Signal>"
  Variant Source/1 -> MATLAB Function2/1(input)
  Real-Imag to Complex1/1 -> Switch1/3  "disrupted_Signal"

== system a2024_V2X_6V_Simulink_model/Subsystem2 ==
  VehicleID : Inport
  Trigger : Inport  Port=2
  busActors3Test1 : Inport  Port=3
  Pilot : Inport  Port=4
  Actors : Inport  Port=5
  Constant2 : Constant  Value=[zeros(19,1)']  SampleTime=-1
  Display : Display
  Entity Multicast1 : EntityMulticast  InputPortMessageModes=m
  Integer to Bit Converter2 : simulink/Logic and Bit Operations/Integer to Bit Converter  nbits=16  signedInputValues=Signed  bitOrder=MSB first  outDtype=boolean
  MATLAB Function1 : MATLAB Function  TreatAsAtomicUnit=on
  OFDM Modulator : commofdm/OFDM Modulator  StatePerturbationForJacobian=1.0e-05  FFTLength=64  NumGuardBandCarriers=[0;0]  InsertDCNull=on  PilotInputPort=on  PilotCarrierIndices=[12; 26; 40; 54]  CyclicPrefixLength=32  Windowing=off  WindowLength=16  OversamplingFactor=3  NumSymbols=1  NumTransmitAntennas=1  SimulateUsing=Interpreted execution
  Rectangular QAM Modulator Baseband2 : commdigbbndam3/Rectangular QAM Modulator Baseband  M=2^6  InType=Bit  Enc=Binary  Mapping=[0:15]  PowType=Average Power  MinDist=2  AvgPow=P_Signal  PeakPow=1  Ph=0  outDtype=double  outWordLen=16  outUDDataType=sfix(16)  outFracLenMode=Best precision  outFracLen=15  outDataTypeStr=double  outLastDataTypeStr=double
      settings: LibrarySourceBlock=|
      | commhdldigbbndam/Rectangular QAM
      | Modulator
      | Baseband
  Send1 : Send  OutputPortMessageModes=m
  To Workspace : ToWorkspace  VariableName=v3  SampleTime=-1
  Vector Concatenate : Concatenate
  VehicleData : Outport
  V3 : Outport  Port=2
  wires:
  MATLAB Function1/1(Actor) -> To Workspace/1, Display/1, Integer to Bit Converter2/1
  Vector Concatenate/1 -> OFDM Modulator/1  "After QAM Mod"
  Send1/1 -> Entity Multicast1/1
  Rectangular QAM Modulator Baseband2/1 -> Vector Concatenate/1
  Constant2/1 -> Vector Concatenate/2
  Actors/1 -> MATLAB Function1/3(EgoData)
  OFDM Modulator/1 -> Send1/1  "OFDM modulated"
  Integer to Bit Converter2/1 -> Rectangular QAM Modulator Baseband2/1
  Trigger/1 -> MATLAB Function1/Trigger
  busActors3Test1/1 -> MATLAB Function1/1(busActors3Test1)
  VehicleID/1 -> MATLAB Function1/2(VehicleID)
  Pilot/1 -> OFDM Modulator/2
  MATLAB Function1/2(VehicleData) -> VehicleData/1
  MATLAB Function1/3(counter) -> V3/1
